simulink model "es2_sim"  (R2023b)
settings: Solver=VariableStepAuto  StartTime=0.0  StopTime=10.0  RelTol=1e-3
values from neighbouring files (symbols this model uses):
  x0 = [3;5]    [es2.m]
settings Model: Creator=stefa  LastModifiedBy=stefa

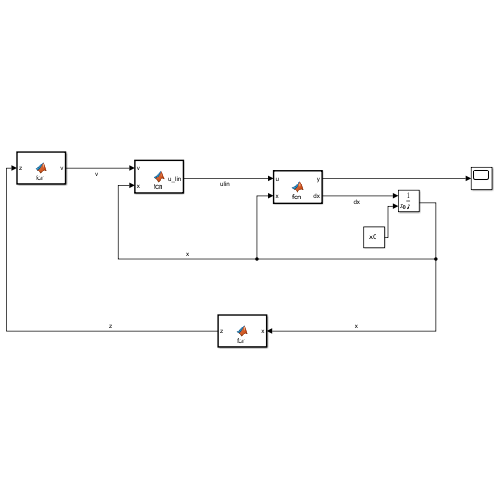
[thumbnail: Simulink's stored preview of the top-level diagram]
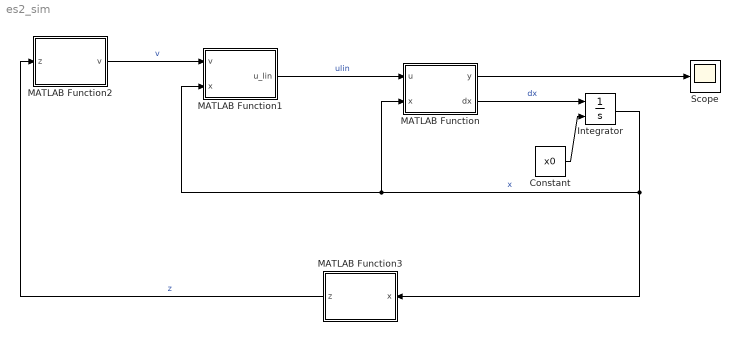
== system es2_sim ==
  Constant : Constant  Value=x0
  Integrator : Integrator  InitialConditionSource=external
  MATLAB Function : MATLAB Function  TreatAsAtomicUnit=on
  MATLAB Function1 : MATLAB Function  TreatAsAtomicUnit=on
  MATLAB Function2 : MATLAB Function  TreatAsAtomicUnit=on
  MATLAB Function3 : MATLAB Function  TreatAsAtomicUnit=on
  Scope : Scope
  wires:
  Constant/1 -> Integrator/2
  MATLAB Function/2(dx) -> Integrator/1  "dx"
  Integrator/1 -> MATLAB Function3/1(x), MATLAB Function1/2(x), MATLAB Function/2(x)  "x"
  MATLAB Function1/1(u_lin) -> MATLAB Function/1(u)  "ulin"
  MATLAB Function2/1(v) -> MATLAB Function1/1(v)  "v"
  MATLAB Function3/1(z) -> MATLAB Function2/1(z)  "z"
  MATLAB Function/1(y) -> Scope/1

== matlab function es2_sim/MATLAB Function ==
  data: u input; y output; x input; dx output
function [y,dx]= fcn(u,x)
x1=x(1);
x2=x(2);
dx=[(x1^2+x1)*x2;
    -4*x2+x1-x2*u+3*u];
y=5*x1;

== matlab function es2_sim/MATLAB Function2 ==
  data: z input; v output
function v = fcn(z)
k=[12.5 7.5];
v=-k(1)*z(1)-k(2)*z(2);

== matlab function es2_sim/MATLAB Function3 ==
  data: x input; z output
function z = fcn(x)
x1=x(1);
x2=x(2);

z=[5*x1; 5*x2*(x1^2 + x1)];

== matlab function es2_sim/MATLAB Function1 ==
  data: v input; u_lin output; x input
function u_lin = fcn(v,x)
x1=x(1);
x2=x(2);
u_lin=((5*x1^2 + 5*x1)*(x1 - 4*x2) - v + 5*x2^2*(2*x1 + 1)*(x1^2 + x1))/((5*x1^2 + 5*x1)*(x2 - 3));
